simulink model "my_spring"  (R2021b)
settings: Solver=FixedStepAuto  StartTime=0.0  StopTime=10.0  RelTol=1e-3
settings Model: Creator=lywan  LastModifiedBy=lywan
settings RTWCC: GenCodeOnly=on  Toolchain=AUTOSAR Adaptive | CMake  TargetLang=C++
settings GRTTargetCC: TargetLangStandard=C++11 (ISO)

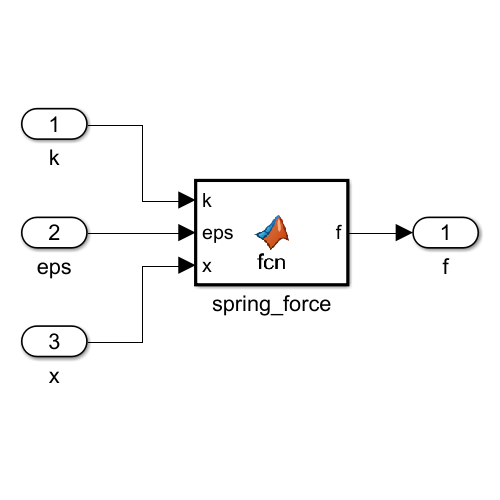
[thumbnail: Simulink's stored preview of the top-level diagram]
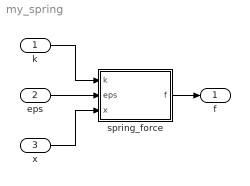
== system my_spring ==
  k : Inport
  eps : Inport  Port=2
  x : Inport  Port=3
  spring_force : MATLAB Function  TreatAsAtomicUnit=on
  f : Outport
  wires:
  k/1 -> spring_force/1(k)
  eps/1 -> spring_force/2(eps)
  x/1 -> spring_force/3(x)
  spring_force/1(f) -> f/1

== matlab function my_spring/spring_force ==
  data: k input; f output; eps input; x input
function f = fcn(k, eps, x)

f = -k*x - eps*x^3;
